simulink model "Mass_spring_sys"  (R2015a)
settings: Solver=ode3  StartTime=0.0  StopTime=200  RelTol=1e-3
values from neighbouring files (symbols this model uses):
  B = [2,5,3,6]    [Lab1.m]    (also in cruise_speed.m = 30; mass_spring.m = 30)
  Fa = 300    [cruise_speed.m]    (also in mass_spring.m; multiple_element_sys.m)
  K = 15    [mass_spring.m]
  M = 750    [cruise_speed.m]    (also in mass_spring.m = 705)
settings Model: Creator=Bilal  LastModifiedBy=Bilal

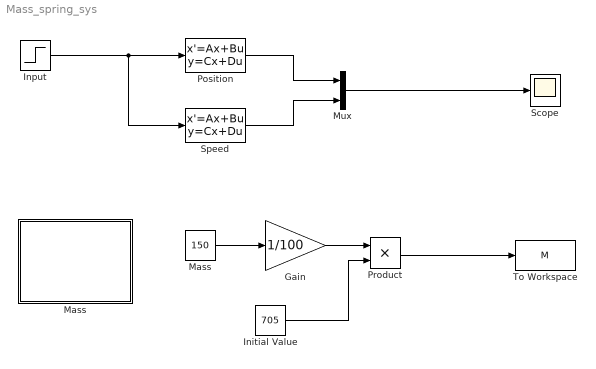
== system Mass_spring_sys ==
  Gain : Gain  Gain=1/100
  "Initial Value " : Constant  Value=705
  "Input " : Step  Time=0  SampleTime=0
  Mass : Constant  Value=150
  "Mass " : Subsystem  DialogController=hmiCreateDDGDialog  IsWebBlock=on  mask(MathWorksWebBlock){webBlockId=5fdcfc05-0b97-48f3-8b39-1a3b10aac9a4, webBlockType=discreteknob, ShowInLibBrowser=on, ShowInitialText=on, HMISrcModelName=Mass_spring_sys}
      mask prompts: webBlockId "WebBlock Id"; webBlockType "WebBlock Type"; HMISrcModelName "Source Model"
      mask Help: helpview([docroot '/mapfiles/simulink.map'], 'hmi_rotary_switch')
      mask Display:
      | model = bdroot(gcb);
      | if strcmp(get_param(model,'BlockDiagramType'), 'library')
      |     image([(matlabroot) '/toolbox/simulink/hmi/icons/DiscreteKnob.png']);
      | end
  Mux : Mux  Inputs=2
  "Position " : StateSpace  A=[0 1;(-K/M) (-B/M)]  B=[0;Fa/M]  C=[1 0]  D=[0]  X0=0  ContinuousStateAttributes='position'
  Product : Product
  Scope : Scope
  "Speed " : StateSpace  A=[0 1;(-K/M) (-B/M)]  B=[0;Fa/M]  C=[0 1]  D=[0]  X0=0  ContinuousStateAttributes='speed'
  To Workspace : ToWorkspace  VariableName=M  SampleTime=-1
      settings: MaxDataPoints=1  Save2DSignal=2-D array (concatenate along first dimension)
  wires:
  "Input "/1 -> "Speed "/1, "Position "/1
  "Speed "/1 -> Mux/2
  "Position "/1 -> Mux/1
  Mux/1 -> Scope/1
  Product/1 -> To Workspace/1
  Gain/1 -> Product/1
  Mass/1 -> Gain/1
  "Initial Value "/1 -> Product/2

== system Mass_spring_sys/Mass  ==
